simulink model "kalmanF1"  (Simulink 8.9)
settings: Solver=FixedStepAuto  StartTime=0.0  StopTime=100.0  FixedStep=0.01  RelTol=1e-3
undefined symbols (not defined in the file): Discrete, Time
libraries: ctrlSharedLib x1, discretizing x1
settings Model: Creator=Soutrik  LastModifiedBy=Soutrik
settings DataIOCC: LimitDataPoints=off  SaveFormat=Dataset  SignalLoggingSaveFormat=Dataset
settings OptimizationCC: LifeSpan=auto
settings DebuggingCC: UnderspecifiedInitializationDetection=Simplified  MergeDetectMultiDrivingBlocksExec=error  FcnCallInpInsideContextMsg=error  StateNameClashWarn=none  SFUnexpectedBacktrackingDiag=error  SFNoUnconditionalDefaultTransitionDiag=error  SFExecutionAtInitializationDiag=warning
settings HardwareCC: ProdBitPerPointer=64  ProdBitPerSizeT=64  ProdBitPerPtrDiffT=64  ProdLargestAtomicFloat=Float  ProdIntDivRoundTo=Zero  ProdEndianess=LittleEndian  ProdWordSize=64  ProdHWDeviceType=Intel->x86-64 (Windows64)
settings ModelReferenceCC: PropagateSignalLabelsOutOfModel=on
settings GRTTargetCC: TargetLangStandard=C99 (ISO)  GeneratePreprocessorConditionals=Use local settings  CombineOutputUpdateFcns=on  GRTInterface=off
settings ConfigComp: CovMetricSettings=dwe  CovHtmlReporting=off  CovSaveCumulativeToWorkspaceVar=off  CovSaveSingleToWorkspaceVar=off  CovExternalEMLEnable=on

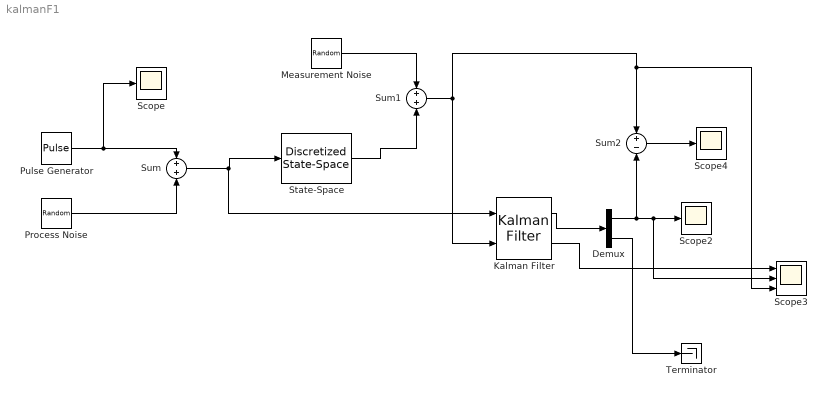
== system kalmanF1 ==
  Demux : Demux  Outputs=2
  Kalman Filter : ctrlSharedLib/Kalman Filter  TimeDomain=Discrete-Time  UseCurrentEstimator=on  ModelSource=Individual A, B, C, D matrices  ModelSourceVariable=ss(0.95,1,1,0,1)  A=[0 1;-1 -0.8]  B=[0;1]  C=[1 0]  D=0  NumberOfStates=1  NumberOfInputs=1  NumberOfOutputs=1  InitialEstimateSource=Dialog  X0=0  P0=10  UseK=off  UseGH=off  NumberOfProcessNoiseInputs=1  G=1  TimeInvariantG=on  H=0  TimeInvariantH=on  Q=diag([0 100])  TimeInvariantQ=on  R=1.25  TimeInvariantR=on  N=0  TimeInvariantN=on  AddInputPort=on  AddEnablePort=off  OutputEstimatedY=off  OutputP=on  Ts=-1
  Measurement Noise : RandomNumber  Variance=0.001  Seed=47  SampleTime=0.01
  Process Noise : RandomNumber  Variance=0.001  Seed=59  SampleTime=0.01
  Pulse Generator : DiscretePulseGenerator  PulseType=Time based  Period=10  PulseWidth=50
  Scope : Scope
  Scope2 : Scope
  Scope3 : Scope  NumInputPorts=3
  Scope4 : Scope
  State-Space : discretizing/Discretized State-Space  A=[0 1;-1 -0.8]  B=[0;1]  C=[1 0]  D=0  ic=0  AbsTol=auto  SampleTime=0.01  method=tustin  Wc=1
  Sum : Sum  Inputs=2
  Sum1 : Sum  Inputs=2
  Sum2 : Sum  Inputs=+-
  Terminator : Terminator
  wires:
  Pulse Generator/1 -> Scope/1, Sum/1
  Process Noise/1 -> Sum/2
  Sum/1 -> Kalman Filter/1, State-Space/1
  Measurement Noise/1 -> Sum1/1
  State-Space/1 -> Sum1/2
  Sum1/1 -> Kalman Filter/2, Scope3/3, Sum2/1
  Kalman Filter/1 -> Demux/1
  Demux/1 -> Scope3/2, Scope2/1, Sum2/2
  Sum2/1 -> Scope4/1
  Demux/2 -> Terminator/1
  Kalman Filter/2 -> Scope3/1
